simulink model "Prescan_Carsim_0118_cs_old"  (R2019b)
settings: Solver=ode5  StartTime=0.0  StopTime=inf  FixedStep=1/1000  RelTol=1e-3
PreLoadFcn:
  | mbxruntime.callbacks.PreLoadFcn(bdroot);
PostLoadFcn:
  | mbxruntime.callbacks.PostLoadFcn(bdroot);
InitFcn:
  | mbxruntime.callbacks.InitFcn(bdroot);
  | Initialization_Func;
  | %T01_Init_2106;
StartFcn:
  | mbxruntime.callbacks.StartFcn(bdroot);
  | current_sys=gcs;
  | speedblock=Simulink.findBlocks(current_sys,'Name','speed_kmh_Gain');
  | h1=add_exec_event_listener(speedblock,'PostOutputs',@SpeedVisulization);
  | outblock=Simulink.findBlocks(current_sys,'Name','trajectorycurveoutput_Gain');
  | CurveTrajectoryListenerHandle=add_exec_event_listener(outblock,'PostOutputs',@TrajectoryCurve_CallBack);
  | lanedatablock=Simulink.findBlocks(current_sys,'Name','LaneData_Gain');
  | CurveLaneListenerHandle=add_exec_event_listener(lanedatablock,'PostOutputs',@CurveLane_CallBack);
StopFcn:
  | mbxruntime.callbacks.StopFcn(bdroot);
model workspace: external: MAT-File .\Prescan_Carsim_0118_cs_hws.mat (data not in the file)
values from neighbouring files (symbols this model uses):
  g = 9.8    [Initialization_Func.m]
  InitialPlanningParameter = [0,0,1,0,2,2,2,40,60]'    [Initialization_Func.m]
  Kf = 20000    [Initialization_Func.m]
  Kr = 20000    [Initialization_Func.m]
  Lr = 1.644    [Initialization_Func.m]
  M = 1275    [Initialization_Func.m]
  nG = 24    [Initialization_Func.m]
  V = 60/3.6    (= 16.6666666667)    [Initialization_Func.m]
  VehicleBaseLength = Lf+Lr    (= 2.66)    [Initialization_Func.m]
undefined symbols (not defined in the file or in its folder): AAx, AAy, AAz, AVx, AVy, AVz, Ax, Ay, Az, canChannel, DiscIntNeverNeededParam, InitialDPMPDF_Comfort, InitialDPMPDF_Efficiency, InitialDPMPDF_Safety, InitialPDF_DEM, mbxruntime, NormalisedTrajectoryIndicator_Pool, Parameter_Indicator_LookUpTable, Prescan_Carsim_1230_cs_0658e9ca1334a8be, Prescan_Carsim_1230_cs_08c5eb9a1bd7376a, Prescan_Carsim_1230_cs_6cfd759b89b9fc85, Prescan_Carsim_1230_cs_9435cc1cceb5050d, Prescan_Carsim_1230_cs_ac716d34d49f74ab, Prescan_Carsim_1230_cs_be02757d7f212dd5, Rational_Coefficient_Learning, SteeringWheel, TrajectoryIndicatorRange, Vx, Vy, Vz, WheelL0, WheelL1, WheelR0, WheelR1
libraries: canmsglib x11, dsparch4 x6, canlib x3, PreScanSimulinkLibrary x3, Solver_SF x1, autolibshared x1
(part 4 of 8)

== system Prescan_Carsim_0118_cs_old/WheelR0_BMW_X5_SUV_1/Actuator/visu_Rotate ==
  In1 : Inport
  sfun_RPYActuator : S-Function  FunctionName=sfun_RPYActuator  Parameters=SParameter1, SParameter2, SampleTime  SFunctionDeploymentMode=off  EnableBusSupport=off  mask(Legacy Function){SFunctionSpec=void prescan_outputFcn(void ** work1,  PRESCAN_XYZ_DATA u1[1]), SParameter1=UniqueID, SParameter2=uint8([Object3DID 0]), SampleTime=TimeStep, ShowSpec=on}
      mask prompts: SParameter1 "P1:"; SParameter2 "P2:"; SampleTime "Sample time (-1 for inherited):"; ShowSpec "Display function specification"
      mask help:
      | This block allows you to call the legacy functions specified by the following Legacy Code Tool definition:
      | def.SFunctionName = 'sfun_PositionActuator';
      | def.OutputFcnSpec = 'void prescan_outputFcn(void ** work1,  PRESCAN_XYZ_DATA u1[1])';
      | def.StartFcnSpec = 'void prescan_startFcn(void ** work1, uint8 p1[], double p2)';
      | def.TerminateFcnSpec = 'void prescan_terminateFcn(void ** work1)';
      | def.HeaderFiles = {'prescan_positionactuator_data.h', 'prescan_header_data.h', 'prescan_SFunLibrary.h', 'prescan_CreateLogHandler.h', 'prescan_CreateErrorHandler.h'};
      | def.SourceFiles = {'prescan_MexLogHandler.cpp', 'prescan_SimStructErrorHandler.cpp', 'prescan_ConcurrentLogHandler.cpp', 'prescan_ConcurrentErrorHandler.cpp'};
      | def.HostLibFiles = {'sensorinterfaced.lib'};
      | def.TargetLibFiles = {'sensorinterfaced.so'};
      | def.IncPaths = {'.', 'C:\prescandev\vislibrary\vis\..\pimp\include\sensors\InterfaceRTW'};
      | def.SrcPaths = {'.'};
      | def.LibPaths = {'C:\\prescandev\\vislibrary_build\lib'};
      | def.SampleTime = 'parameterized';
      mask Help: <p>This block was generated automatically by the Legacy Code Tool. For detailed help on this tool, call<a href="matlab:legacy_code('help')"> legacy_code('help')</a>.</p>
      mask Callback ShowSpec:
      | if strcmp(get_param(gcbh, 'ShowSpec'), 'on')
      |   set_param(gcbh, 'MaskDisplay', sprintf('fprintf(''%s'');', get_param(gcbh, 'SFunctionSpec')));
      | else
      |   set_param(gcbh, 'MaskDisplay', sprintf('fprintf(''%s'');', get_param(gcbh, 'FunctionName')));
      | end
      mask Display: fprintf('void prescan_outputFcn(void ** work1,  PRESCAN_XYZ_DATA u1[1])');
  wires:
  In1/1 -> sfun_RPYActuator/1

== system Prescan_Carsim_0118_cs_old/WheelR0_BMW_X5_SUV_1/Actuator/visu_Translate ==
  In1 : Inport
  sfun_PositionActuator : S-Function  FunctionName=sfun_PositionActuator  Parameters=SParameter1, SParameter2, SampleTime  SFunctionDeploymentMode=off  EnableBusSupport=off  mask(Legacy Function){SFunctionSpec=void prescan_outputFcn(void ** work1,  PRESCAN_XYZ_DATA u1[1]), SParameter1=uint8([Object3DID 0]), SParameter2=UniqueID, SampleTime=TimeStep, ShowSpec=on}
      mask prompts: SParameter1 "P1:"; SParameter2 "P2:"; SampleTime "Sample time (-1 for inherited):"; ShowSpec "Display function specification"
      mask help:
      | This block allows you to call the legacy functions specified by the following Legacy Code Tool definition:
      | def.SFunctionName = 'sfun_PositionActuator';
      | def.OutputFcnSpec = 'void prescan_outputFcn(void ** work1,  PRESCAN_XYZ_DATA u1[1])';
      | def.StartFcnSpec = 'void prescan_startFcn(void ** work1, uint8 p1[], double p2)';
      | def.TerminateFcnSpec = 'void prescan_terminateFcn(void ** work1)';
      | def.HeaderFiles = {'prescan_positionactuator_data.h', 'prescan_header_data.h', 'prescan_SFunLibrary.h', 'prescan_CreateLogHandler.h', 'prescan_CreateErrorHandler.h'};
      | def.SourceFiles = {'prescan_MexLogHandler.cpp', 'prescan_SimStructErrorHandler.cpp', 'prescan_ConcurrentLogHandler.cpp', 'prescan_ConcurrentErrorHandler.cpp'};
      | def.HostLibFiles = {'sensorinterfaced.lib'};
      | def.TargetLibFiles = {'sensorinterfaced.so'};
      | def.IncPaths = {'.', 'C:\prescandev\vislibrary\vis\..\pimp\include\sensors\InterfaceRTW'};
      | def.SrcPaths = {'.'};
      | def.LibPaths = {'C:\\prescandev\\vislibrary_build\lib'};
      | def.SampleTime = 'parameterized';
      mask Help: <p>This block was generated automatically by the Legacy Code Tool. For detailed help on this tool, call<a href="matlab:legacy_code('help')"> legacy_code('help')</a>.</p>
      mask Callback ShowSpec:
      | if strcmp(get_param(gcbh, 'ShowSpec'), 'on')
      |   set_param(gcbh, 'MaskDisplay', sprintf('fprintf(''%s'');', get_param(gcbh, 'SFunctionSpec')));
      | else
      |   set_param(gcbh, 'MaskDisplay', sprintf('fprintf(''%s'');', get_param(gcbh, 'FunctionName')));
      | end
      mask Display: fprintf('void prescan_outputFcn(void ** work1,  PRESCAN_XYZ_DATA u1[1])');
  wires:
  In1/1 -> sfun_PositionActuator/1

== system Prescan_Carsim_0118_cs_old/WheelR1_BMW_X5_SUV_1/Actuator/visu_Rotate ==
  In1 : Inport
  sfun_RPYActuator : S-Function  FunctionName=sfun_RPYActuator  Parameters=SParameter1, SParameter2, SampleTime  SFunctionDeploymentMode=off  EnableBusSupport=off  mask(Legacy Function){SFunctionSpec=void prescan_outputFcn(void ** work1,  PRESCAN_XYZ_DATA u1[1]), SParameter1=UniqueID, SParameter2=uint8([Object3DID 0]), SampleTime=TimeStep, ShowSpec=on}
      mask prompts: SParameter1 "P1:"; SParameter2 "P2:"; SampleTime "Sample time (-1 for inherited):"; ShowSpec "Display function specification"
      mask help:
      | This block allows you to call the legacy functions specified by the following Legacy Code Tool definition:
      | def.SFunctionName = 'sfun_PositionActuator';
      | def.OutputFcnSpec = 'void prescan_outputFcn(void ** work1,  PRESCAN_XYZ_DATA u1[1])';
      | def.StartFcnSpec = 'void prescan_startFcn(void ** work1, uint8 p1[], double p2)';
      | def.TerminateFcnSpec = 'void prescan_terminateFcn(void ** work1)';
      | def.HeaderFiles = {'prescan_positionactuator_data.h', 'prescan_header_data.h', 'prescan_SFunLibrary.h', 'prescan_CreateLogHandler.h', 'prescan_CreateErrorHandler.h'};
      | def.SourceFiles = {'prescan_MexLogHandler.cpp', 'prescan_SimStructErrorHandler.cpp', 'prescan_ConcurrentLogHandler.cpp', 'prescan_ConcurrentErrorHandler.cpp'};
      | def.HostLibFiles = {'sensorinterfaced.lib'};
      | def.TargetLibFiles = {'sensorinterfaced.so'};
      | def.IncPaths = {'.', 'C:\prescandev\vislibrary\vis\..\pimp\include\sensors\InterfaceRTW'};
      | def.SrcPaths = {'.'};
      | def.LibPaths = {'C:\\prescandev\\vislibrary_build\lib'};
      | def.SampleTime = 'parameterized';
      mask Help: <p>This block was generated automatically by the Legacy Code Tool. For detailed help on this tool, call<a href="matlab:legacy_code('help')"> legacy_code('help')</a>.</p>
      mask Callback ShowSpec:
      | if strcmp(get_param(gcbh, 'ShowSpec'), 'on')
      |   set_param(gcbh, 'MaskDisplay', sprintf('fprintf(''%s'');', get_param(gcbh, 'SFunctionSpec')));
      | else
      |   set_param(gcbh, 'MaskDisplay', sprintf('fprintf(''%s'');', get_param(gcbh, 'FunctionName')));
      | end
      mask Display: fprintf('void prescan_outputFcn(void ** work1,  PRESCAN_XYZ_DATA u1[1])');
  wires:
  In1/1 -> sfun_RPYActuator/1

== system Prescan_Carsim_0118_cs_old/WheelR1_BMW_X5_SUV_1/Actuator/visu_Translate ==
  In1 : Inport
  sfun_PositionActuator : S-Function  FunctionName=sfun_PositionActuator  Parameters=SParameter1, SParameter2, SampleTime  SFunctionDeploymentMode=off  EnableBusSupport=off  mask(Legacy Function){SFunctionSpec=void prescan_outputFcn(void ** work1,  PRESCAN_XYZ_DATA u1[1]), SParameter1=uint8([Object3DID 0]), SParameter2=UniqueID, SampleTime=TimeStep, ShowSpec=on}
      mask prompts: SParameter1 "P1:"; SParameter2 "P2:"; SampleTime "Sample time (-1 for inherited):"; ShowSpec "Display function specification"
      mask help:
      | This block allows you to call the legacy functions specified by the following Legacy Code Tool definition:
      | def.SFunctionName = 'sfun_PositionActuator';
      | def.OutputFcnSpec = 'void prescan_outputFcn(void ** work1,  PRESCAN_XYZ_DATA u1[1])';
      | def.StartFcnSpec = 'void prescan_startFcn(void ** work1, uint8 p1[], double p2)';
      | def.TerminateFcnSpec = 'void prescan_terminateFcn(void ** work1)';
      | def.HeaderFiles = {'prescan_positionactuator_data.h', 'prescan_header_data.h', 'prescan_SFunLibrary.h', 'prescan_CreateLogHandler.h', 'prescan_CreateErrorHandler.h'};
      | def.SourceFiles = {'prescan_MexLogHandler.cpp', 'prescan_SimStructErrorHandler.cpp', 'prescan_ConcurrentLogHandler.cpp', 'prescan_ConcurrentErrorHandler.cpp'};
      | def.HostLibFiles = {'sensorinterfaced.lib'};
      | def.TargetLibFiles = {'sensorinterfaced.so'};
      | def.IncPaths = {'.', 'C:\prescandev\vislibrary\vis\..\pimp\include\sensors\InterfaceRTW'};
      | def.SrcPaths = {'.'};
      | def.LibPaths = {'C:\\prescandev\\vislibrary_build\lib'};
      | def.SampleTime = 'parameterized';
      mask Help: <p>This block was generated automatically by the Legacy Code Tool. For detailed help on this tool, call<a href="matlab:legacy_code('help')"> legacy_code('help')</a>.</p>
      mask Callback ShowSpec:
      | if strcmp(get_param(gcbh, 'ShowSpec'), 'on')
      |   set_param(gcbh, 'MaskDisplay', sprintf('fprintf(''%s'');', get_param(gcbh, 'SFunctionSpec')));
      | else
      |   set_param(gcbh, 'MaskDisplay', sprintf('fprintf(''%s'');', get_param(gcbh, 'FunctionName')));
      | end
      mask Display: fprintf('void prescan_outputFcn(void ** work1,  PRESCAN_XYZ_DATA u1[1])');
  wires:
  In1/1 -> sfun_PositionActuator/1

== system Prescan_Carsim_0118_cs_old/BMW_X5_SUV_1/DEM updating and Preference Estimation/UpdateDEM/Construct Comparison Group ==
  FeedBack_FromDriver : Inport
  TrajectoryIndicator : Inport  Port=2
  Comparison Group_1 : MATLAB Function  TreatAsAtomicUnit=on
  Constant : Constant  Value=NormalisedTrajectoryIndicator_Pool
  Constant7 : Constant  Value=TrajectoryIndicatorRange
  FeedBack : Outport
  Query_Normalized : Outport  Port=2
  Evaluated_NormlisedTrajectoryIndicator : Outport  Port=3
  LastPreference_Normalised : Outport  Port=4
  wires:
  Comparison Group_1/2(Query_Compare) -> Query_Normalized/1
  FeedBack_FromDriver/1 -> Comparison Group_1/1(Feedback_Driver)
  TrajectoryIndicator/1 -> Comparison Group_1/2(Real_Trajectory_Indicator)
  Constant7/1 -> Comparison Group_1/3(TrajectoryIndicatorRange)
  Constant/1 -> Comparison Group_1/4(NormalisedTrajectoryIndicator_Pool)
  Comparison Group_1/1(FeedBack) -> FeedBack/1
  Comparison Group_1/3(Evaluated_NormalisedTrajectoryIndicator) -> Evaluated_NormlisedTrajectoryIndicator/1
  Comparison Group_1/4(LastPreference_Normalised) -> LastPreference_Normalised/1

== system Prescan_Carsim_0118_cs_old/BMW_X5_SUV_1/DEM updating and Preference Estimation/UpdateDEM/Online DEM updating ==
  FeedBack : Inport
  Query_Compare : Inport  Port=2
  PriorPDF_DEM : Inport  Port=3
  PriorDPMPDF_Safety : Inport  Port=4
  PriorDPMPDF_Comfort : Inport  Port=5
  PriorDPMPDF_Efficiency : Inport  Port=6
  Evaluated_Normalised : Inport  Port=7
  LastPreference_NormalisedTrajectoryIndicator : Inport  Port=8
  Constant : Constant  Value=NormalisedTrajectoryIndicator_Pool
  Constant3 : Constant  Value=Rational_Coefficient_Learning
  "Select the Next Trajectory " : MATLAB Function  TreatAsAtomicUnit=on
  UPdate DEM : MATLAB Function  TreatAsAtomicUnit=on
  Next_ExpectedTrajectoryIndicator : Outport
  Next_ExpectedTrajectoryID : Outport  Port=2
  wires:
  FeedBack/1 -> UPdate DEM/1(FeedBack)
  Query_Compare/1 -> UPdate DEM/2(Query)
  PriorPDF_DEM/1 -> UPdate DEM/3(PriorPDF_DEM)
  PriorDPMPDF_Safety/1 -> UPdate DEM/4(PriorDPMPDF_Safety)
  PriorDPMPDF_Comfort/1 -> UPdate DEM/5(PriorDPMPDF_Comfort)
  PriorDPMPDF_Efficiency/1 -> UPdate DEM/6(PriorDPMPDF_Efficiency)
  Constant3/1 -> "Select the Next Trajectory "/8(Rational_Coefficient_Learning), UPdate DEM/7(Rational_Coefficient_Learning)
  UPdate DEM/1(PostPDF_DEM) -> "Select the Next Trajectory "/1(PriorPDF_DEM)
  UPdate DEM/2(PostDPMPDF_Safety) -> "Select the Next Trajectory "/2(PriorDPMPDF_Safety)
  UPdate DEM/3(PostDPMPDF_Comfort) -> "Select the Next Trajectory "/3(PriorDPMPDF_Comfort)
  UPdate DEM/4(PostDPMPDF_Effociency) -> "Select the Next Trajectory "/4(PriorDPMPDF_Efficiency)
  "Select the Next Trajectory "/2(ExpectedNext_QueryID) -> Next_ExpectedTrajectoryID/1
  "Select the Next Trajectory "/1(ExpectedNext_NormalisedTrajectoryIndicator) -> Next_ExpectedTrajectoryIndicator/1
  Constant/1 -> "Select the Next Trajectory "/5(NormalisedTrajectoryIndicator_Pool)
  Evaluated_Normalised/1 -> "Select the Next Trajectory "/6(Evaluated_NormalisedTrajectoryIndicator)
  LastPreference_NormalisedTrajectoryIndicator/1 -> "Select the Next Trajectory "/7(LastPreference_NormalisedTrajectoryIndicator)

== system Prescan_Carsim_0118_cs_old/BMW_X5_SUV_1/DEM updating and Preference Estimation/UpdateDEM/Trajectory Planning Parameter Management1 ==
  Expected_TrajectoryIndicators : Inport
  ExpectedNext_QueryID : Inport  Port=2
  Constant : Constant  Value=InitialPlanningParameter
  Constant4 : Constant  Value=Parameter_Indicator_LookUpTable
  Determine planning parameter according to the expected TrajectoryIndicators_LookUpTable : MATLAB Function  TreatAsAtomicUnit=on
  From : From  Commented=on  GotoTag=Parameter_Indicator_LookUpTable  TagVisibility=global
  From2 : From  Commented=on  GotoTag=InitialPlanningParameter  TagVisibility=global
  Trajectory parameter : Outport
  wires:
  Expected_TrajectoryIndicators/1 -> Determine planning parameter according to the expected TrajectoryIndicators_LookUpTable/2(unused)
  ExpectedNext_QueryID/1 -> Determine planning parameter according to the expected TrajectoryIndicators_LookUpTable/3(ExpectedNext_QueryID)
  Determine planning parameter according to the expected TrajectoryIndicators_LookUpTable/1(PlanningParameter) -> Trajectory parameter/1
  Constant/1 -> Determine planning parameter according to the expected TrajectoryIndicators_LookUpTable/1(IntialTrajectoryPlanningParameter)
  Constant4/1 -> Determine planning parameter according to the expected TrajectoryIndicators_LookUpTable/4(Parameter_IndicatorLookUpTable)

== system Prescan_Carsim_0118_cs_old/BMW_X5_SUV_1/DEM updating and Preference Estimation/UpdateDEM/Trajectory Planning Parameter Management2 ==
  Expected_TrajectoryIndicators : Inport
  Next_ExpectedTrajectoryIndicatorID : Inport  Port=2
  Constant4 : Constant  Value=Parameter_Indicator_LookUpTable
  Determine planning parameter according to the expected TrajectoryIndicators_LookUpTable : MATLAB Function  TreatAsAtomicUnit=on
  Trajectory parameter : Outport
  wires:
  Expected_TrajectoryIndicators/1 -> Determine planning parameter according to the expected TrajectoryIndicators_LookUpTable/1(unused)
  Next_ExpectedTrajectoryIndicatorID/1 -> Determine planning parameter according to the expected TrajectoryIndicators_LookUpTable/2(ExpectedNext_QueryID)
  Determine planning parameter according to the expected TrajectoryIndicators_LookUpTable/1(PlanningParameter) -> Trajectory parameter/1
  Constant4/1 -> Determine planning parameter according to the expected TrajectoryIndicators_LookUpTable/3(Parameter_IndicatorLookUpTable)

== system Prescan_Carsim_0118_cs_old/BMW_X5_SUV_1/DEM updating and Preference Estimation/UpdateDEM/online DPM building preference estimation accordign to feedback ==
  note: DEM-
      | Update the DEM and Estimate the Preference
  feedback : Inport
  Trajectory_Indicators : Inport  Port=2
  " Driver Perception Model preference to trajectory indicator" : Subsystem  Commented=on
  Constant : Constant  Value=NormalisedTrajectoryIndicator_Pool
  Constant1 : Constant  Value=InitialPDF_DEM
      settings: AttributesFormatString=|
      | The Initial probability density Distribution
      | of the S-C-E weight of the DEM
  Constant2 : Constant  Value=InitialDPMPDF_Safety
      settings: AttributesFormatString=|
      | The Initial probability density Distribution
      | of the DPM for S-C-E
  Constant3 : Constant  Value=Rational_Coefficient_Learning
  Constant5 : Constant  Value=InitialDPMPDF_Comfort
      settings: AttributesFormatString=|
      | The Initial probability density Distribution
      | of the DPM for S-C-E
  Constant6 : Constant  Value=InitialDPMPDF_Efficiency
      settings: AttributesFormatString=|
      | The Initial probability density Distribution
      | of the DPM for S-C-E
  Constant7 : Constant  Value=TrajectoryIndicatorRange
  MATLAB Function : MATLAB Function  TreatAsAtomicUnit=on
  Terminator{,1..3} (4 alike) : Terminator
  Expected_TrajectoryIndicators : Outport
  ExpectedNext_QueryID : Outport  Port=2
  wires:
  MATLAB Function/1(ExpectedNext_NormalisedTrajectoryIndicator) -> Expected_TrajectoryIndicators/1
  MATLAB Function/2(ExpectedNext_QueryID) -> ExpectedNext_QueryID/1
  MATLAB Function/6(PostDPMPDF_Effociency) -> Terminator3/1
  MATLAB Function/5(PostDPMPDF_Comfort) -> Terminator2/1
  Constant7/1 -> MATLAB Function/8(TrajectoryIndicatorRange)
  Constant6/1 -> MATLAB Function/7(InitialDPMPDF_Efficiency)
  Constant5/1 -> MATLAB Function/6(InitialDPMPDF_Comfort)
  MATLAB Function/4(PostDPMPDF_Safety) -> Terminator1/1
  MATLAB Function/3(PostPDF_DEM) -> Terminator/1
  Trajectory_Indicators/1 -> MATLAB Function/2(Real_Trajectory_Indicator)
  Constant3/1 -> MATLAB Function/9(Rational_Coefficient_Learning)
  Constant2/1 -> MATLAB Function/5(InitialDPMPDF_Safety)
  Constant1/1 -> MATLAB Function/4(InitialPDF_DEM)
  Constant/1 -> MATLAB Function/3(NormalisedTrajectoryIndicator_Pool)
  feedback/1 -> MATLAB Function/1(FeedBack)

== system Prescan_Carsim_0118_cs_old/BMW_X5_SUV_1/DriverFeedBack/Generate the FeedBack Obtainment Trigger Signal/Subsystem ==
  In1 : Inport
  Trigger : TriggerPort  TriggerType=falling  VariantControl=Variant  PortDimensions=1
  Beginning Time : Outport
  wires:
  In1/1 -> Beginning Time/1

== system Prescan_Carsim_0118_cs_old/BMW_X5_SUV_1/SELF_Demux/compas converter/cart2compas ==
  Angle [deg] : Inport
  Constant : Constant  Value=90
  Constant1 : Constant  Value=360
  Gain : Gain  Gain=1/360
  Gain1 : Gain  Gain=360
  Gain2 : Gain  Gain=-1
  Rounding Function : Rounding
  Sum : Sum  Inputs=|-+
  Sum1 : Sum  Inputs=-+|
  Sum2 : Sum  Inputs=++|
  heading [deg] : Outport
  wires:
  Gain/1 -> Rounding Function/1
  Rounding Function/1 -> Gain1/1
  Gain1/1 -> Sum/1
  Angle [deg]/1 -> Sum1/2
  Sum/1 -> Gain2/1
  Sum1/1 -> Gain/1, Sum/2
  Constant/1 -> Sum1/1
  Gain2/1 -> Sum2/2
  Constant1/1 -> Sum2/1
  Sum2/1 -> heading [deg]/1

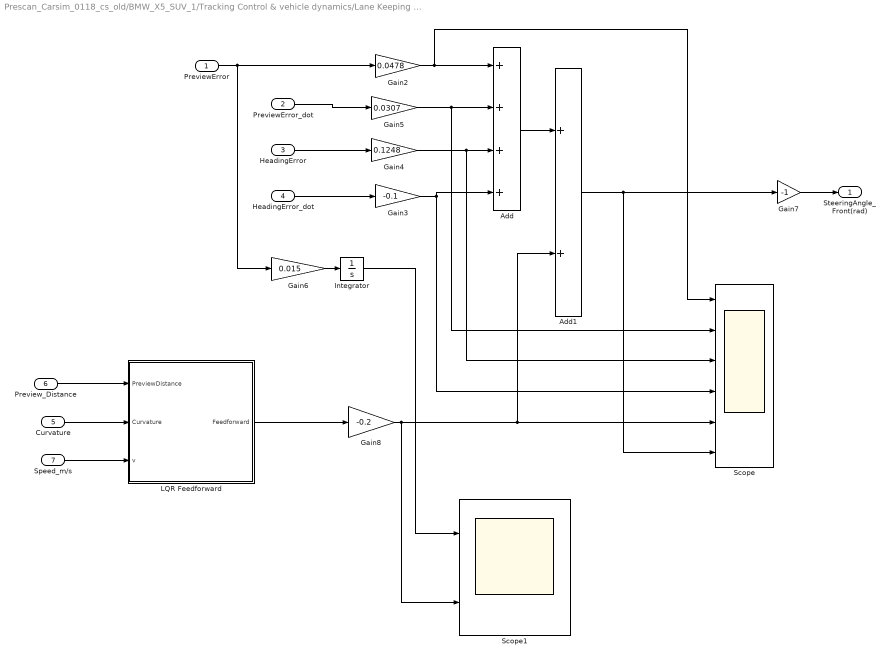
== system Prescan_Carsim_0118_cs_old/BMW_X5_SUV_1/Tracking Control & vehicle dynamics/Lane Keeping Assistance/Path Tracking - LQR controller ==
  PreviewError : Inport
  PreviewError_dot : Inport  Port=2
  HeadingError : Inport  Port=3
  HeadingError_dot : Inport  Port=4
  Curvature : Inport  Port=5
  Preview_Distance : Inport  Port=6
  Speed_m/s : Inport  Port=7
  Add : Sum  Inputs=++++
  Add1 : Sum
  Gain2 : Gain  Gain=0.0478
  Gain3 : Gain  Gain=-0.1
  Gain4 : Gain  Gain=0.1248
  Gain5 : Gain  Gain=0.0307
  Gain6 : Gain  Gain=0.015
  Gain7 : Gain  Gain=-1
  Gain8 : Gain  Gain=-0.2
  Integrator : Integrator
  LQR Feedforward : MATLAB Function  TreatAsAtomicUnit=on
  Scope : Scope  NumInputPorts=6
  Scope1 : Scope  NumInputPorts=2
  SteeringAngle_Front(rad) : Outport
  wires:
  PreviewError/1 -> Gain6/1, Gain2/1
  Gain4/1 -> Scope/3, Add/3
  Gain5/1 -> Scope/2, Add/2
  Gain3/1 -> Scope/4, Add/4
  Gain8/1 -> Scope/5, Add1/2, Scope1/2
  Gain2/1 -> Scope/1, Add/1
  Gain7/1 -> SteeringAngle_Front(rad)/1
  Add/1 -> Add1/1
  HeadingError_dot/1 -> Gain3/1
  Add1/1 -> Scope/6, Gain7/1
  Gain6/1 -> Integrator/1
  PreviewError_dot/1 -> Gain5/1
  HeadingError/1 -> Gain4/1
  Preview_Distance/1 -> LQR Feedforward/1(PreviewDistance)
  LQR Feedforward/1(Feedforward) -> Gain8/1
  Curvature/1 -> LQR Feedforward/2(Curvature)
  Integrator/1 -> Scope1/1
  Speed_m/s/1 -> LQR Feedforward/3(v)

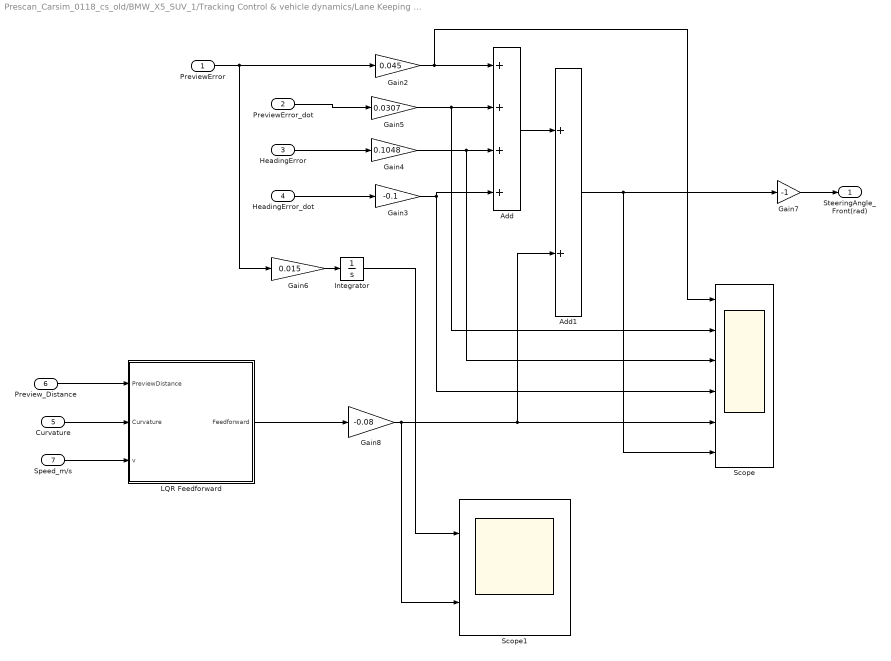
== system Prescan_Carsim_0118_cs_old/BMW_X5_SUV_1/Tracking Control & vehicle dynamics/Lane Keeping Assistance/Path Tracking - LQR controller1 ==
  PreviewError : Inport
  PreviewError_dot : Inport  Port=2
  HeadingError : Inport  Port=3
  HeadingError_dot : Inport  Port=4
  Curvature : Inport  Port=5
  Preview_Distance : Inport  Port=6
  Speed_m/s : Inport  Port=7
  Add : Sum  Inputs=++++
  Add1 : Sum
  Gain2 : Gain  Gain=0.045
  Gain3 : Gain  Gain=-0.1
  Gain4 : Gain  Gain=0.1048
  Gain5 : Gain  Gain=0.0307
  Gain6 : Gain  Gain=0.015
  Gain7 : Gain  Gain=-1
  Gain8 : Gain  Gain=-0.08
  Integrator : Integrator
  LQR Feedforward : MATLAB Function  TreatAsAtomicUnit=on
  Scope : Scope  NumInputPorts=6
  Scope1 : Scope  NumInputPorts=2
  SteeringAngle_Front(rad) : Outport
  wires:
  PreviewError/1 -> Gain6/1, Gain2/1
  Gain4/1 -> Scope/3, Add/3
  Gain5/1 -> Scope/2, Add/2
  Gain3/1 -> Scope/4, Add/4
  Gain8/1 -> Scope/5, Add1/2, Scope1/2
  Gain2/1 -> Scope/1, Add/1
  Gain7/1 -> SteeringAngle_Front(rad)/1
  Add/1 -> Add1/1
  HeadingError_dot/1 -> Gain3/1
  Add1/1 -> Scope/6, Gain7/1
  Gain6/1 -> Integrator/1
  PreviewError_dot/1 -> Gain5/1
  HeadingError/1 -> Gain4/1
  Preview_Distance/1 -> LQR Feedforward/1(PreviewDistance)
  LQR Feedforward/1(Feedforward) -> Gain8/1
  Curvature/1 -> LQR Feedforward/2(Curvature)
  Integrator/1 -> Scope1/1
  Speed_m/s/1 -> LQR Feedforward/3(v)

== system Prescan_Carsim_0118_cs_old/BMW_X5_SUV_1/Tracking Control & vehicle dynamics/Lane Keeping Assistance/SMC characters ==
  note: 双移线和直线
  Abs : Abs
  Constant1 : Constant  Value=3.2
  Constant15 : Constant  Value=0.5
  Constant17 : Constant  Value=0.4
  Constant18 : Constant  Value=1.5
  Demux : Demux
  Display : Display
  Mux : Mux
  Mux1 : Mux
  Switch : Switch  Criteria=u2 > Threshold  Threshold=0.4
  st_angle_max10 : Constant  Value=3.5
  st_angle_max7 : Constant  Value=0.03
  st_angle_max8 : Constant  Value=2.3
  st_angle_max9 : Constant  Value=0.12
  tag scope: SMC_c1=global, SMC_c2=global, delta=global, kapa=global
  wires:
  Demux/1 -> [SMC_c1], Display/1
  st_angle_max7/1 -> Mux/3
  Constant18/1 -> Mux/1
  Demux/3 -> [delta]
  Mux/1 -> Switch/1
  [Lateral_Offset] -> Abs/1
  Demux/4 -> [kapa]
  Switch/1 -> Demux/1
  Constant1/1 -> Mux1/1
  Constant15/1 -> Mux/2
  Demux/2 -> [SMC_c2]
  st_angle_max9/1 -> Mux1/3
  Abs/1 -> Switch/2
  st_angle_max8/1 -> Mux/4
  st_angle_max10/1 -> Mux1/4
  Constant17/1 -> Mux1/2
  Mux1/1 -> Switch/3

== system Prescan_Carsim_0118_cs_old/BMW_X5_SUV_1/Tracking Control & vehicle dynamics/Lane Keeping Assistance/derivative_filter ==
  In1 : Inport
  Gain1 : Gain  Gain=0.8
  Gain2 : Gain  Gain=50
  Integrator2 : Integrator
  Sum1 : Sum  Inputs=|+-
  Out1 : Outport
  wires:
  Sum1/1 -> Gain2/1
  Integrator2/1 -> Sum1/2
  Gain1/1 -> Out1/1
  Gain2/1 -> Gain1/1, Integrator2/1
  In1/1 -> Sum1/1

== system Prescan_Carsim_0118_cs_old/BMW_X5_SUV_1/Tracking Control & vehicle dynamics/Lane Keeping Assistance/derivative_filter  ==
  In1 : Inport
  Gain1 : Gain  Gain=0.42
  Gain2 : Gain  Gain=40
  Integrator2 : Integrator
  Saturation : Saturate  UpperLimit=4  LowerLimit=-4
  Sum1 : Sum  Inputs=|+-
  Out1 : Outport
  wires:
  Saturation/1 -> Out1/1
  In1/1 -> Sum1/1
  Gain2/1 -> Integrator2/1, Gain1/1
  Integrator2/1 -> Sum1/2
  Sum1/1 -> Gain2/1
  Gain1/1 -> Saturation/1

== system Prescan_Carsim_0118_cs_old/BMW_X5_SUV_1/trajectory planning/A substitution for the above trajectory planning subsystem/Trajectory Planning For Curve under beginning-global ==
  note: The trajectory is a DataArray with 3 columns, the first two is the (X,Y) coordinates of the planed path ( under the vehicle coordinates system) , the third column is the planned velocity of that path point.
  RoadLane_Plan : Inport
  Parameter_TrajectoryPlan : Inport  Port=2
  VehicleWidth : Inport  Port=3
  LaneWidth : Inport  Port=4
  VehicleState_Global : Inport  Port=5
  Enable : EnablePort  PropagateVarSize=During execution
  Trigger : TriggerPort  VariantControl=Variant  PortDimensions=1
  LaneData_Gain2 : Gain
  Trajectory Planning For Curve : MATLAB Function  TreatAsAtomicUnit=on
  Path Plan : Outport
  Speed_Planned_kmh : Outport  Port=2
  PlanPathDataLength : Outport  Port=3
  VehicleState_CurvePlanningBeginning : Outport  Port=4  InitialOutput=[0 0 0]
  wires:
  Trajectory Planning For Curve/3(PlanPathDataLength_Curve) -> PlanPathDataLength/1
  LaneWidth/1 -> Trajectory Planning For Curve/4(LaneWidth)
  VehicleWidth/1 -> Trajectory Planning For Curve/3(VehicleWidth)
  VehicleState_Global/1 -> VehicleState_CurvePlanningBeginning/1
  RoadLane_Plan/1 -> LaneData_Gain2/1
  Trajectory Planning For Curve/1(Path_Plan) -> Path Plan/1
  Trajectory Planning For Curve/2(Speed_Planned_kmh) -> Speed_Planned_kmh/1
  Parameter_TrajectoryPlan/1 -> Trajectory Planning For Curve/2(Parameter_TrajectoryPlan)
  LaneData_Gain2/1 -> Trajectory Planning For Curve/1(RoadLane_Plan)

== system Prescan_Carsim_0118_cs_old/BMW_X5_SUV_1/trajectory planning/Specific Curve Trajectory Planning/Trajectory Planning For Curve under beginning-global ==
  note: The trajectory is a DataArray with 3 columns, the first two is the (X,Y) coordinates of the planed path ( under the vehicle coordinates system) , the third column is the planned velocity of that path point.
  RoadLane_Plan : Inport
  Parameter_TrajectoryPlan : Inport  Port=2
  VehicleWidth : Inport  Port=3
  LaneWidth : Inport  Port=4
  VehicleState_Global : Inport  Port=5
  Trigger : TriggerPort  VariantControl=Variant  InitialTriggerSignalState=negative  PortDimensions=1
  LaneData_Gain : Gain
  Subsystem : Subsystem  Commented=on
  Trajectory Planning For Curve : MATLAB Function  TreatAsAtomicUnit=on
  Path Plan : Outport
  Speed_Planned_kmh : Outport  Port=2
  PlanPathDataLength : Outport  Port=3
  wires:
  Trajectory Planning For Curve/3(PlanPathDataLength_Curve) -> PlanPathDataLength/1
  LaneWidth/1 -> Subsystem/4(In4), Trajectory Planning For Curve/4(LaneWidth)
  VehicleWidth/1 -> Subsystem/3(In3), Trajectory Planning For Curve/3(VehicleWidth)
  VehicleState_Global/1 -> Trajectory Planning For Curve/5(VehicleState_Beginning)
  Trajectory Planning For Curve/2(Speed_Planned_kmh) -> Speed_Planned_kmh/1
  Parameter_TrajectoryPlan/1 -> Subsystem/2(In2), Trajectory Planning For Curve/2(Parameter_TrajectoryPlan)
  RoadLane_Plan/1 -> LaneData_Gain/1
  Trajectory Planning For Curve/1(PathPlan_Global) -> Path Plan/1
  LaneData_Gain/1 -> Subsystem/1(In1), Trajectory Planning For Curve/1(RoadLane_Plan)

== system Prescan_Carsim_0118_cs_old/BMW_X5_SUV_1/trajectory planning/Subsystem/Determination of Curve Road No ==
  Determine Curve No According the vehicle position : MATLAB Function  TreatAsAtomicUnit=on
      settings: AttributesFormatString=Curve 1:curve_length+60(30 meters befor and after curve)
  Curve No : Outport
  wires:
  [VehicleState_Global] -> Determine Curve No According the vehicle position/1(VehicleState_Global)
  Determine Curve No According the vehicle position/1(Curve_No) -> Curve No/1

== system Prescan_Carsim_0118_cs_old/BMW_X5_SUV_1/DEM updating and Preference Estimation/UpdateDEM/online DPM building preference estimation accordign to feedback/ Driver Perception Model preference to trajectory indicator ==
  "preference estimation " : Inport
  "Next Trajectory Sample Indicators " : Subsystem
  trajectory indicators : Outport
  wires:
  "preference estimation "/1 -> "Next Trajectory Sample Indicators "/1(In1)
  "Next Trajectory Sample Indicators "/1(Out1) -> trajectory indicators/1

== system Prescan_Carsim_0118_cs_old/BMW_X5_SUV_1/trajectory planning/Specific Curve Trajectory Planning/Trajectory Planning For Curve under beginning-global/Subsystem ==
  In1 : Inport
  In2 : Inport  Port=2
  In3 : Inport  Port=3
  In4 : Inport  Port=4
  Curvature Mode Solve : Subsystem
  Heading Mode Solve : Subsystem
  Length Mode Solve : Subsystem
  MATLAB Function : MATLAB Function  TreatAsAtomicUnit=on
  Path Planning_OSQP Transformation : MATLAB Function  TreatAsAtomicUnit=on
  Path merging and Speed OSQP Transformation : MATLAB Function  TreatAsAtomicUnit=on
  Path planning3 : Subsystem
  Terminator : Terminator
  Out1 : Outport
  Out2 : Outport  Port=2
  Out3 : Outport  Port=3
  Out4 : Outport  Port=4
  Out5 : Outport  Port=5
  Out6 : Outport  Port=6
  wires:
  Path merging and Speed OSQP Transformation/5(Speedlp) -> Path planning3/1(lp)
  Path Planning_OSQP Transformation/2(mode2_Curveture) -> Curvature Mode Solve/1(mode)
  Path Planning_OSQP Transformation/1(mode_Length) -> Length Mode Solve/1(mode)
  Curvature Mode Solve/1(path_alpha) -> Path merging and Speed OSQP Transformation/2(alpha_curvature)
  Path Planning_OSQP Transformation/3(mode4_HeadingError) -> Heading Mode Solve/1(mode)
  MATLAB Function/1(RoadLaneBorder_ForPlan) -> Path merging and Speed OSQP Transformation/3(RoadLaneBorder_ForPlan), Path Planning_OSQP Transformation/1(RoadLaneBorder_ForPlan)
  Length Mode Solve/1(Length_alpha) -> Path merging and Speed OSQP Transformation/1(alpha_path_length)
  In4/1 -> MATLAB Function/3(LaneWidth)
  Heading Mode Solve/1(Heading_alpha) -> Terminator/1
  In1/1 -> MATLAB Function/1(RoadLane_Plan)
  In3/1 -> MATLAB Function/2(VehicleWidth)
  In2/1 -> Path merging and Speed OSQP Transformation/4(Parameter_PathPlan)
  Path merging and Speed OSQP Transformation/4(pathInterpY) -> Out5/1
  MATLAB Function/2(Num_LanePlan) -> Out3/1
  Path planning3/1(speed) -> Out6/1
  Path merging and Speed OSQP Transformation/2(pathPolyY) -> Out2/1
  Path merging and Speed OSQP Transformation/1(pathPolyX) -> Out1/1
  Path merging and Speed OSQP Transformation/3(pathInterpX) -> Out4/1

== system Prescan_Carsim_0118_cs_old/BMW_X5_SUV_1/DEM updating and Preference Estimation/UpdateDEM/online DPM building preference estimation accordign to feedback/ Driver Perception Model preference to trajectory indicator/Next Trajectory Sample Indicators  ==
  In1 : Inport
  Out1 : Outport
  wires:
  In1/1 -> Out1/1

== system Prescan_Carsim_0118_cs_old/BMW_X5_SUV_1/trajectory planning/Specific Curve Trajectory Planning/Trajectory Planning For Curve under beginning-global/Subsystem/Curvature Mode Solve ==
  mode : Inport
  Bus Selector : BusSelector  OutputSignals=m,n,P_nnz,P_x,P_i,P_p,q,A_nnz,A_x,A_i,A_p,l,u
  Bus Selector1 : BusSelector  OutputSignals=m,n,P_nnz,P_x,P_i,P_p,q,A_nnz,A_x,A_i,A_p,l,u
  Display{,1..13} (14 alike) : Display
  Terminator : Terminator
  Terminator1 : Terminator
  osqpcec : S-Function  FunctionName=osqpcec  SFunctionDeploymentMode=off  EnableBusSupport=off  mask(Legacy Function){SFunctionSpec=int32 y3 = qpSolver(int32 u1, int32 u2, int32 u3, double u4[], int32 u5[], int32 u6[],double u7[], int32 u8, double u9[], int32 u10[], int32 u11[],double u12[], double u13[], double y1[1000], double y2[1000]), ShowSpec=off}
      mask prompts: ShowSpec "Display function specification"
      mask help:
      | This block allows you to call the legacy functions specified by the following Legacy Code Tool definition:
      | def.SFunctionName = 'osqpcec';
      | def.OutputFcnSpec = 'int32 y3 = qpSolver(int32 u1, int32 u2, int32 u3, double u4[], int32 u5[], int32 u6[],double u7[], int32 u8, double u9[], int32 u10[], int32 u11[],double u12[], double u13[], double y1[1000], double y2[1000])';
      | def.HeaderFiles = {'osqpcec03xiataokai.h', 'util.h', 'types.h', 'scaling.h', 'proj.h', 'polish.h', 'osqp_configure.h', 'osqp.h', 'lin_sys.h', 'lin_alg.h', 'kkt.h', 'glob_opts.h', 'error.h', 'ctrlc.h', 'cs.h', 'auxil.h'};
      | def.SourceFiles = {'osqpcec03xiataokai.cpp'};
      | def.HostLibFiles = {'libosqp.a'};
      | def.IncPaths = {'./test03/h'};
      | def.SrcPaths = {'./test03/cpp'};
      | def.LibPaths = {'./test03/lib'};
      mask Help: <p>This block was generated automatically by the Legacy Code Tool. For detailed help on this tool, call<a href="matlab:legacy_code('help')"> legacy_code('help')</a>.</p>
      mask Callback ShowSpec:
      | if strcmp(get_param(gcbh, 'ShowSpec'), 'on')
      |   set_param(gcbh, 'MaskDisplay', sprintf('fprintf(''%s'');', get_param(gcbh, 'SFunctionSpec')));
      | else
      |   set_param(gcbh, 'MaskDisplay', sprintf('fprintf(''%s'');', get_param(gcbh, 'FunctionName')));
      | end
      mask Display: fprintf('osqpcec');
  path_alpha : Outport
  wires:
  Bus Selector/2 -> Display1/1  "<n>"
  Bus Selector/5 -> Display4/1  "<P_i>"
  Bus Selector/11 -> Display10/1  "<A_p>"
  Bus Selector/7 -> Display6/1  "<q>"
  Bus Selector/4 -> Display3/1  "<P_x>"
  Bus Selector/10 -> Display9/1  "<A_i>"
  Bus Selector/8 -> Display7/1  "<A_nnz>"
  Bus Selector/1 -> Display/1  "<m>"
  Bus Selector/9 -> Display8/1  "<A_x>"
  Bus Selector/13 -> Display12/1  "<u>"
  Bus Selector/6 -> Display5/1  "<P_p>"
  Bus Selector/12 -> Display11/1  "<l>"
  Bus Selector/3 -> Display2/1  "<P_nnz>"
  mode/1 -> Bus Selector1/1, Bus Selector/1
  Bus Selector1/10 -> osqpcec/10  "<A_i>"
  Bus Selector1/13 -> osqpcec/13  "<u>"
  Bus Selector1/9 -> osqpcec/9  "<A_x>"
  Bus Selector1/7 -> osqpcec/7  "<q>"
  Bus Selector1/8 -> osqpcec/8  "<A_nnz>"
  Bus Selector1/3 -> osqpcec/3  "<P_nnz>"
  Bus Selector1/4 -> osqpcec/4  "<P_x>"
  Bus Selector1/1 -> osqpcec/1  "<m>"
  Bus Selector1/5 -> osqpcec/5  "<P_i>"
  Bus Selector1/2 -> osqpcec/2  "<n>"
  Bus Selector1/12 -> osqpcec/12  "<l>"
  Bus Selector1/11 -> osqpcec/11  "<A_p>"
  Bus Selector1/6 -> osqpcec/6  "<P_p>"
  osqpcec/1 -> path_alpha/1, Display13/1  "x"
  osqpcec/2 -> Terminator/1  "y"
  osqpcec/3 -> Terminator1/1  "return"

== system Prescan_Carsim_0118_cs_old/BMW_X5_SUV_1/trajectory planning/Specific Curve Trajectory Planning/Trajectory Planning For Curve under beginning-global/Subsystem/Heading Mode Solve ==
  mode : Inport
  Bus Selector : BusSelector  OutputSignals=m,n,P_nnz,P_x,P_i,P_p,q,A_nnz,A_x,A_i,A_p,l,u
  Bus Selector1 : BusSelector  OutputSignals=m,n,P_nnz,P_x,P_i,P_p,q,A_nnz,A_x,A_i,A_p,l,u
  Display{,1..13} (14 alike) : Display
  Terminator : Terminator
  Terminator1 : Terminator
  osqpcec : S-Function  FunctionName=osqpcec  SFunctionDeploymentMode=off  EnableBusSupport=off  mask(Legacy Function){SFunctionSpec=int32 y3 = qpSolver(int32 u1, int32 u2, int32 u3, double u4[], int32 u5[], int32 u6[],double u7[], int32 u8, double u9[], int32 u10[], int32 u11[],double u12[], double u13[], double y1[1000], double y2[1000]), ShowSpec=off}
      mask prompts: ShowSpec "Display function specification"
      mask help:
      | This block allows you to call the legacy functions specified by the following Legacy Code Tool definition:
      | def.SFunctionName = 'osqpcec';
      | def.OutputFcnSpec = 'int32 y3 = qpSolver(int32 u1, int32 u2, int32 u3, double u4[], int32 u5[], int32 u6[],double u7[], int32 u8, double u9[], int32 u10[], int32 u11[],double u12[], double u13[], double y1[1000], double y2[1000])';
      | def.HeaderFiles = {'osqpcec03xiataokai.h', 'util.h', 'types.h', 'scaling.h', 'proj.h', 'polish.h', 'osqp_configure.h', 'osqp.h', 'lin_sys.h', 'lin_alg.h', 'kkt.h', 'glob_opts.h', 'error.h', 'ctrlc.h', 'cs.h', 'auxil.h'};
      | def.SourceFiles = {'osqpcec03xiataokai.cpp'};
      | def.HostLibFiles = {'libosqp.a'};
      | def.IncPaths = {'./test03/h'};
      | def.SrcPaths = {'./test03/cpp'};
      | def.LibPaths = {'./test03/lib'};
      mask Help: <p>This block was generated automatically by the Legacy Code Tool. For detailed help on this tool, call<a href="matlab:legacy_code('help')"> legacy_code('help')</a>.</p>
      mask Callback ShowSpec:
      | if strcmp(get_param(gcbh, 'ShowSpec'), 'on')
      |   set_param(gcbh, 'MaskDisplay', sprintf('fprintf(''%s'');', get_param(gcbh, 'SFunctionSpec')));
      | else
      |   set_param(gcbh, 'MaskDisplay', sprintf('fprintf(''%s'');', get_param(gcbh, 'FunctionName')));
      | end
      mask Display: fprintf('osqpcec');
  Heading_alpha : Outport
  wires:
  Bus Selector/2 -> Display1/1  "<n>"
  Bus Selector/5 -> Display4/1  "<P_i>"
  Bus Selector/11 -> Display10/1  "<A_p>"
  Bus Selector/7 -> Display6/1  "<q>"
  Bus Selector/4 -> Display3/1  "<P_x>"
  Bus Selector/10 -> Display9/1  "<A_i>"
  Bus Selector/8 -> Display7/1  "<A_nnz>"
  Bus Selector/1 -> Display/1  "<m>"
  Bus Selector/9 -> Display8/1  "<A_x>"
  Bus Selector/13 -> Display12/1  "<u>"
  Bus Selector/6 -> Display5/1  "<P_p>"
  Bus Selector/12 -> Display11/1  "<l>"
  Bus Selector/3 -> Display2/1  "<P_nnz>"
  mode/1 -> Bus Selector1/1, Bus Selector/1
  Bus Selector1/10 -> osqpcec/10  "<A_i>"
  Bus Selector1/13 -> osqpcec/13  "<u>"
  Bus Selector1/9 -> osqpcec/9  "<A_x>"
  Bus Selector1/7 -> osqpcec/7  "<q>"
  Bus Selector1/8 -> osqpcec/8  "<A_nnz>"
  Bus Selector1/3 -> osqpcec/3  "<P_nnz>"
  Bus Selector1/4 -> osqpcec/4  "<P_x>"
  Bus Selector1/1 -> osqpcec/1  "<m>"
  Bus Selector1/5 -> osqpcec/5  "<P_i>"
  Bus Selector1/2 -> osqpcec/2  "<n>"
  Bus Selector1/12 -> osqpcec/12  "<l>"
  Bus Selector1/11 -> osqpcec/11  "<A_p>"
  Bus Selector1/6 -> osqpcec/6  "<P_p>"
  osqpcec/1 -> Heading_alpha/1, Display13/1  "x"
  osqpcec/2 -> Terminator/1  "y"
  osqpcec/3 -> Terminator1/1  "return"

== system Prescan_Carsim_0118_cs_old/BMW_X5_SUV_1/trajectory planning/Specific Curve Trajectory Planning/Trajectory Planning For Curve under beginning-global/Subsystem/Length Mode Solve ==
  mode : Inport
  Bus Selector : BusSelector  OutputSignals=m,n,P_nnz,P_x,P_i,P_p,q,A_nnz,A_x,A_i,A_p,l,u
  Bus Selector1 : BusSelector  OutputSignals=m,n,P_nnz,P_x,P_i,P_p,q,A_nnz,A_x,A_i,A_p,l,u
  Display{,1..13} (14 alike) : Display
  Terminator : Terminator
  Terminator1 : Terminator
  osqpcec : S-Function  FunctionName=osqpcec  SFunctionDeploymentMode=off  EnableBusSupport=off  mask(Legacy Function){SFunctionSpec=int32 y3 = qpSolver(int32 u1, int32 u2, int32 u3, double u4[], int32 u5[], int32 u6[],double u7[], int32 u8, double u9[], int32 u10[], int32 u11[],double u12[], double u13[], double y1[1000], double y2[1000]), ShowSpec=off}
      mask prompts: ShowSpec "Display function specification"
      mask help:
      | This block allows you to call the legacy functions specified by the following Legacy Code Tool definition:
      | def.SFunctionName = 'osqpcec';
      | def.OutputFcnSpec = 'int32 y3 = qpSolver(int32 u1, int32 u2, int32 u3, double u4[], int32 u5[], int32 u6[],double u7[], int32 u8, double u9[], int32 u10[], int32 u11[],double u12[], double u13[], double y1[1000], double y2[1000])';
      | def.HeaderFiles = {'osqpcec03xiataokai.h', 'util.h', 'types.h', 'scaling.h', 'proj.h', 'polish.h', 'osqp_configure.h', 'osqp.h', 'lin_sys.h', 'lin_alg.h', 'kkt.h', 'glob_opts.h', 'error.h', 'ctrlc.h', 'cs.h', 'auxil.h'};
      | def.SourceFiles = {'osqpcec03xiataokai.cpp'};
      | def.HostLibFiles = {'libosqp.a'};
      | def.IncPaths = {'./test03/h'};
      | def.SrcPaths = {'./test03/cpp'};
      | def.LibPaths = {'./test03/lib'};
      mask Help: <p>This block was generated automatically by the Legacy Code Tool. For detailed help on this tool, call<a href="matlab:legacy_code('help')"> legacy_code('help')</a>.</p>
      mask Callback ShowSpec:
      | if strcmp(get_param(gcbh, 'ShowSpec'), 'on')
      |   set_param(gcbh, 'MaskDisplay', sprintf('fprintf(''%s'');', get_param(gcbh, 'SFunctionSpec')));
      | else
      |   set_param(gcbh, 'MaskDisplay', sprintf('fprintf(''%s'');', get_param(gcbh, 'FunctionName')));
      | end
      mask Display: fprintf('osqpcec');
  Length_alpha : Outport
  wires:
  Bus Selector/2 -> Display1/1  "<n>"
  Bus Selector/5 -> Display4/1  "<P_i>"
  Bus Selector/11 -> Display10/1  "<A_p>"
  Bus Selector/7 -> Display6/1  "<q>"
  Bus Selector/4 -> Display3/1  "<P_x>"
  Bus Selector/10 -> Display9/1  "<A_i>"
  Bus Selector/8 -> Display7/1  "<A_nnz>"
  Bus Selector/1 -> Display/1  "<m>"
  Bus Selector/9 -> Display8/1  "<A_x>"
  Bus Selector/13 -> Display12/1  "<u>"
  Bus Selector/6 -> Display5/1  "<P_p>"
  Bus Selector/12 -> Display11/1  "<l>"
  Bus Selector/3 -> Display2/1  "<P_nnz>"
  mode/1 -> Bus Selector1/1, Bus Selector/1
  Bus Selector1/10 -> osqpcec/10  "<A_i>"
  Bus Selector1/13 -> osqpcec/13  "<u>"
  Bus Selector1/9 -> osqpcec/9  "<A_x>"
  Bus Selector1/7 -> osqpcec/7  "<q>"
  Bus Selector1/8 -> osqpcec/8  "<A_nnz>"
  Bus Selector1/3 -> osqpcec/3  "<P_nnz>"
  Bus Selector1/4 -> osqpcec/4  "<P_x>"
  Bus Selector1/1 -> osqpcec/1  "<m>"
  Bus Selector1/5 -> osqpcec/5  "<P_i>"
  Bus Selector1/2 -> osqpcec/2  "<n>"
  Bus Selector1/12 -> osqpcec/12  "<l>"
  Bus Selector1/11 -> osqpcec/11  "<A_p>"
  Bus Selector1/6 -> osqpcec/6  "<P_p>"
  osqpcec/1 -> Length_alpha/1, Display13/1  "x"
  osqpcec/2 -> Terminator/1  "y"
  osqpcec/3 -> Terminator1/1  "return"

== system Prescan_Carsim_0118_cs_old/BMW_X5_SUV_1/trajectory planning/Specific Curve Trajectory Planning/Trajectory Planning For Curve under beginning-global/Subsystem/Path planning3 ==
  lp : Inport
  Bus Selector : BusSelector  OutputSignals=m,n,P_nnz,P_x,P_i,P_p,q,A_nnz,A_x,A_i,A_p,l,u
  Bus Selector1 : BusSelector  OutputSignals=m,n,P_nnz,P_x,P_i,P_p,q,A_nnz,A_x,A_i,A_p,l,u
  Display{,1..13} (14 alike) : Display
  Terminator : Terminator
  Terminator1 : Terminator
  osqpcec : S-Function  FunctionName=osqpcec  SFunctionDeploymentMode=off  EnableBusSupport=off  mask(Legacy Function){SFunctionSpec=int32 y3 = qpSolver(int32 u1, int32 u2, int32 u3, double u4[], int32 u5[], int32 u6[],double u7[], int32 u8, double u9[], int32 u10[], int32 u11[],double u12[], double u13[], double y1[1000], double y2[1000]), ShowSpec=off}
      mask prompts: ShowSpec "Display function specification"
      mask help:
      | This block allows you to call the legacy functions specified by the following Legacy Code Tool definition:
      | def.SFunctionName = 'osqpcec';
      | def.OutputFcnSpec = 'int32 y3 = qpSolver(int32 u1, int32 u2, int32 u3, double u4[], int32 u5[], int32 u6[],double u7[], int32 u8, double u9[], int32 u10[], int32 u11[],double u12[], double u13[], double y1[1000], double y2[1000])';
      | def.HeaderFiles = {'osqpcec03xiataokai.h', 'util.h', 'types.h', 'scaling.h', 'proj.h', 'polish.h', 'osqp_configure.h', 'osqp.h', 'lin_sys.h', 'lin_alg.h', 'kkt.h', 'glob_opts.h', 'error.h', 'ctrlc.h', 'cs.h', 'auxil.h'};
      | def.SourceFiles = {'osqpcec03xiataokai.cpp'};
      | def.HostLibFiles = {'libosqp.a'};
      | def.IncPaths = {'./test03/h'};
      | def.SrcPaths = {'./test03/cpp'};
      | def.LibPaths = {'./test03/lib'};
      mask Help: <p>This block was generated automatically by the Legacy Code Tool. For detailed help on this tool, call<a href="matlab:legacy_code('help')"> legacy_code('help')</a>.</p>
      mask Callback ShowSpec:
      | if strcmp(get_param(gcbh, 'ShowSpec'), 'on')
      |   set_param(gcbh, 'MaskDisplay', sprintf('fprintf(''%s'');', get_param(gcbh, 'SFunctionSpec')));
      | else
      |   set_param(gcbh, 'MaskDisplay', sprintf('fprintf(''%s'');', get_param(gcbh, 'FunctionName')));
      | end
      mask Display: fprintf('osqpcec');
  speed : Outport
  wires:
  Bus Selector/2 -> Display1/1  "<n>"
  Bus Selector/5 -> Display4/1  "<P_i>"
  Bus Selector/11 -> Display10/1  "<A_p>"
  Bus Selector/7 -> Display6/1  "<q>"
  Bus Selector/4 -> Display3/1  "<P_x>"
  Bus Selector/10 -> Display9/1  "<A_i>"
  Bus Selector/8 -> Display7/1  "<A_nnz>"
  Bus Selector/1 -> Display/1  "<m>"
  Bus Selector/9 -> Display8/1  "<A_x>"
  Bus Selector/13 -> Display12/1  "<u>"
  Bus Selector/6 -> Display5/1  "<P_p>"
  Bus Selector/12 -> Display11/1  "<l>"
  Bus Selector/3 -> Display2/1  "<P_nnz>"
  lp/1 -> Bus Selector1/1, Bus Selector/1
  Bus Selector1/10 -> osqpcec/10  "<A_i>"
  Bus Selector1/13 -> osqpcec/13  "<u>"
  Bus Selector1/9 -> osqpcec/9  "<A_x>"
  Bus Selector1/7 -> osqpcec/7  "<q>"
  Bus Selector1/8 -> osqpcec/8  "<A_nnz>"
  Bus Selector1/3 -> osqpcec/3  "<P_nnz>"
  Bus Selector1/4 -> osqpcec/4  "<P_x>"
  Bus Selector1/1 -> osqpcec/1  "<m>"
  Bus Selector1/5 -> osqpcec/5  "<P_i>"
  Bus Selector1/2 -> osqpcec/2  "<n>"
  Bus Selector1/12 -> osqpcec/12  "<l>"
  Bus Selector1/11 -> osqpcec/11  "<A_p>"
  Bus Selector1/6 -> osqpcec/6  "<P_p>"
  osqpcec/1 -> speed/1, Display13/1  "x"
  osqpcec/2 -> Terminator/1  "y"
  osqpcec/3 -> Terminator1/1  "return"
